simulink model "UAM_Flight_control"  (R2024b)
settings: Solver=FixedStepAuto  StartTime=0.0  StopTime=inf  RelTol=1e-3  EnableMultiTasking=on
undefined symbols (not defined in the file): CityMission, control, controlParams, ControlSampleTime, Cruise_a, DiscIntNeverNeededParam, Earth, FixedWingMission, flightState, FSState, FWControlParams, FWTrimSpeed, HoverMission, params, position, R_WAYPOINTTRANSITION, TransitionMission, uavParam, Vt, w_trim, WGS84, zGround
libraries: slpidlib x56, simulink x32, uavalgslib x7, robotcorelib x2, simulink_extras x2, mspfiltlib x1, aerolibtransform2 x1
(part 2 of 13)

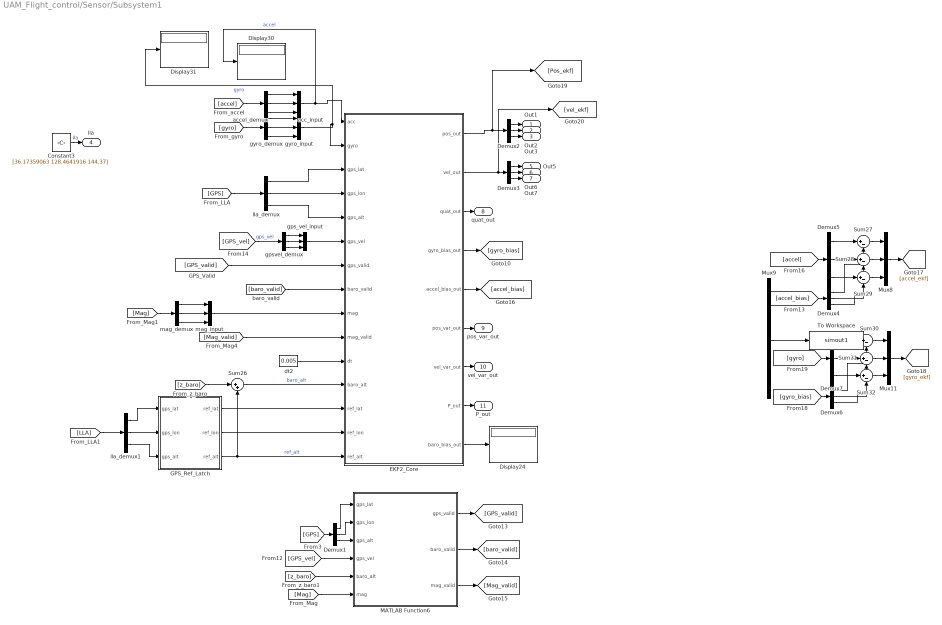
== system UAM_Flight_control/Sensor/Subsystem1 ==
  Constant3 : Constant  Value=[36.17359063 128.4641916 144.37]
  Demux{1..7} (7 alike) : Demux  Outputs=3
  Display24 : Display
  Display30 : Display
  Display31 : Display
  EKF2_Core : Subsystem
  GPS_Ref_Latch : MATLAB Function  TreatAsAtomicUnit=on
  MATLAB Function6 : MATLAB Function  TreatAsAtomicUnit=on
  Mux11 : Mux  Inputs=3
  Mux8 : Mux  Inputs=3
  Mux9 : Mux  Inputs=8
  Sum26 : Sum  Inputs=|++
  Sum{27..32} (6 alike) : Sum  Inputs=|+-
  To Workspace : ToWorkspace  VariableName=simout1  SaveFormat=Structure With Time  SampleTime=-1
  acc_input : Mux  Inputs=3
  accel_demux : Demux  Outputs=3
  dt2 : Constant  Value=0.005
  gps_vel_input : Mux  Inputs=3
  gpsvel_demux : Demux  Outputs=3
  gyro_demux : Demux  Outputs=3
  gyro_input : Mux  Inputs=3
  lla_demux : Demux  Outputs=3
  lla_demux1 : Demux  Outputs=3
  mag_demux : Demux  Outputs=3
  mag_input : Mux  Inputs=3
  Out1 : Outport
  Out2 : Outport  Port=2
  Out3 : Outport  Port=3
  lla : Outport  Port=4
  Out5 : Outport  Port=5
  Out6 : Outport  Port=6
  Out7 : Outport  Port=7
  quat_out : Outport  Port=8
  pos_var_out : Outport  Port=9
  vel_var_out : Outport  Port=10
  P_out : Outport  Port=11
  wires:
  GPS_Ref_Latch/1(ref_lat) -> EKF2_Core/13(ref_lat)
  [Mag] -> MATLAB Function6/6(mag)
  [GPS_vel] -> MATLAB Function6/4(gps_vel)
  EKF2_Core/3(quat_out) -> quat_out/1
  gpsvel_demux/3 -> gps_vel_input/3
  [Mag] -> mag_demux/1
  lla_demux1/3 -> GPS_Ref_Latch/3(gps_alt)
  acc_input/1 -> Display30/1, EKF2_Core/1(acc)  "accel"
  [accel] -> accel_demux/1
  GPS_Ref_Latch/3(ref_alt) -> Sum26/2, EKF2_Core/15(ref_alt)  "ref_alt"
  gyro_demux/3 -> gyro_input/3
  mag_demux/1 -> mag_input/1
  Sum26/1 -> EKF2_Core/12(baro_alt)  "baro_alt"
  gyro_demux/1 -> gyro_input/1
  EKF2_Core/7(vel_var_out) -> vel_var_out/1
  Demux1/2 -> MATLAB Function6/2(gps_lon)
  mag_input/1 -> EKF2_Core/9(mag)
  EKF2_Core/9(baro_bias_out) -> Display24/1
  [baro_valid] -> EKF2_Core/8(baro_valid)
  [LLA] -> lla_demux1/1
  EKF2_Core/5(accel_bias_out) -> [accel_bias]
  Demux2/3 -> Out3/1
  [gyro] -> gyro_demux/1
  MATLAB Function6/1(gps_valid) -> [GPS_valid]
  Demux2/2 -> Out2/1
  [z_baro] -> MATLAB Function6/5(baro_alt)
  [GPS_vel] -> gpsvel_demux/1  "gps_vel"
  gpsvel_demux/1 -> gps_vel_input/1
  Demux2/1 -> Out1/1
  GPS_Ref_Latch/2(ref_lon) -> EKF2_Core/14(ref_lon)
  lla_demux1/1 -> GPS_Ref_Latch/1(gps_lat)
  gyro_demux/2 -> gyro_input/2
  mag_demux/2 -> mag_input/2
  lla_demux/1 -> EKF2_Core/3(gps_lat)
  MATLAB Function6/2(baro_valid) -> [baro_valid]
  [GPS] -> lla_demux/1
  accel_demux/3 -> acc_input/3
  Demux1/1 -> MATLAB Function6/1(gps_lat)
  Demux1/3 -> MATLAB Function6/3(gps_alt)
  MATLAB Function6/3(mag_valid) -> [Mag_valid]
  dt2/1 -> EKF2_Core/11(dt)
  [Mag_valid] -> EKF2_Core/10(mag_valid)
  EKF2_Core/6(pos_var_out) -> pos_var_out/1
  Demux3/2 -> Out6/1
  [z_baro] -> Sum26/1
  accel_demux/1 -> acc_input/1
  [GPS_valid] -> EKF2_Core/7(gps_valid)
  EKF2_Core/2(vel_out) -> [vel_ekf], Demux3/1
  Constant3/1 -> lla/1  "lla"
  lla_demux1/2 -> GPS_Ref_Latch/2(gps_lon)
  gps_vel_input/1 -> EKF2_Core/6(gps_vel)
  accel_demux/2 -> acc_input/2
  gyro_input/1 -> EKF2_Core/2(gyro), Display31/1  "gyro"
  [GPS] -> Demux1/1
  lla_demux/3 -> EKF2_Core/5(gps_alt)
  EKF2_Core/1(pos_out) -> [Pos_ekf], Demux2/1
  EKF2_Core/8(P_out) -> P_out/1
  EKF2_Core/4(gyro_bias_out) -> [gyro_bias]
  lla_demux/2 -> EKF2_Core/4(gps_lon)
  gpsvel_demux/2 -> gps_vel_input/2
  mag_demux/3 -> mag_input/3
  Demux3/3 -> Out7/1
  Demux3/1 -> Out5/1
  Sum31/1 -> Mux11/2
  Demux6/3 -> Sum32/2
  Mux11/1 -> [gyro_ekf]
  [gyro] -> Demux7/1
  Mux8/1 -> [accel_ekf]
  Sum30/1 -> Mux11/1
  Sum29/1 -> Mux8/3
  Sum28/1 -> Mux8/2
  Demux5/1 -> Sum27/1
  Mux9/1 -> To Workspace/1
  Demux6/1 -> Sum30/2
  Demux7/1 -> Sum30/1
  [accel_bias] -> Demux4/1
  Demux7/2 -> Sum31/1
  [gyro_bias] -> Demux6/1
  [accel] -> Demux5/1
  Demux4/2 -> Sum28/2
  Demux5/2 -> Sum28/1
  Demux7/3 -> Sum32/1
  Demux4/3 -> Sum29/2
  Sum27/1 -> Mux8/1
  Sum32/1 -> Mux11/3
  Demux4/1 -> Sum27/2
  Demux6/2 -> Sum31/2
  Demux5/3 -> Sum29/1

== system UAM_Flight_control/Sensor/Subsystem2 ==
  fcc : Inport
  In2 : Inport  Port=2
  Constant1 : Constant  Value=0
  Gain : Gain  Gain=pi/180
  Gain1 : Gain  Gain=pi/180
  Matrix Concatenate : Concatenate  NumInputs=3  Mode=Multidimensional array  ConcatenateDimension=2
  Product{,1..3} (4 alike) : Product
  Trigonometric Function : Trigonometry
  Trigonometric Function1 : Trigonometry  Operator=cos
  Trigonometric Function2 : Trigonometry  Operator=cos
  Trigonometric Function3 : Trigonometry
  Unary Minus{,1..5} (6 alike) : UnaryMinus
  Vector Concatenate : Concatenate  NumInputs=3
  Vector Concatenate1 : Concatenate  NumInputs=3
  Vector Concatenate2 : Concatenate  NumInputs=3
  Out1 : Outport
  wires:
  Product3/1 -> Unary Minus3/1
  Vector Concatenate/1 -> Matrix Concatenate/1
  Trigonometric Function1/1 -> Vector Concatenate1/2, Product3/2, Product/2, Product2/2
  Unary Minus4/1 -> Vector Concatenate2/3
  Vector Concatenate2/1 -> Matrix Concatenate/3
  Trigonometric Function3/1 -> Unary Minus5/1, Product1/2
  Trigonometric Function/1 -> Product1/1, Unary Minus4/1, Product/1
  Gain/1 -> Trigonometric Function2/1, Trigonometric Function/1
  Product/1 -> Unary Minus/1
  Vector Concatenate1/1 -> Matrix Concatenate/2
  Trigonometric Function2/1 -> Product2/1, Product3/1, Vector Concatenate/3
  fcc/1 -> Gain/1
  Gain1/1 -> Trigonometric Function1/1, Trigonometric Function3/1
  Constant1/1 -> Vector Concatenate1/3
  Unary Minus5/1 -> Vector Concatenate1/1
  In2/1 -> Gain1/1
  Unary Minus2/1 -> Vector Concatenate2/1
  Product2/1 -> Unary Minus2/1
  Product1/1 -> Unary Minus1/1
  Unary Minus/1 -> Vector Concatenate/1
  Unary Minus1/1 -> Vector Concatenate/2
  Unary Minus3/1 -> Vector Concatenate2/2
  Matrix Concatenate/1 -> Out1/1

== system UAM_Flight_control/Controller/Auto1/Blend Scheduler ==
  note: Forward Transition Tilt Mode Manager
  FlightMode : Inport
  States : Inport  Port=2
  MixerCommands : Inport  Port=3
  BTalpha : Subsystem  TreatAsAtomicUnit=on
  Bus Creator : BusCreator  Inputs=5
  Bus Selector1 : BusSelector  OutputSignals=w_phi,w_theta,w_psi,w_z
  Constant : Constant  Value=flightState.Transition
  Constant2 : Constant  Value=0.25*uavParam.geom.mass*9.81
  Constant3 : Constant  Value=FWTrimSpeed
  Constant4 : Constant  Value=FWTrimSpeed
  Constant5 : Constant
  Constant6 : Constant  Value=78.54
  Constant7 : Constant
  Demux : Demux
  FTalpha : Subsystem
  Gain3 : Gain  Gain=0
  Mux : Mux
  Product1 : Product
  Product2 : Product
  Product3 : Product
  Relational Operator : RelationalOperator  Operator===  OutDataTypeStr=boolean  RndMeth=Simplest  InputSameDT=off
  Subtract : Sum  Inputs=+-
  Subtract1 : Sum  Inputs=+-
  Sum1 : Sum  Inputs=|++
  Sum3 : Sum  Inputs=|+-
  Switch : Switch  Criteria=u2 > Threshold  SaturateOnIntegerOverflow=off  InputSameDT=off
  Switch1 : Switch  Criteria=u2 > Threshold  SaturateOnIntegerOverflow=off  InputSameDT=off
  MotorCommands : Outport
  alpha : Outport  Port=2
  FlightState : Outport  Port=3
  wires:
  FlightMode/1 -> Relational Operator/1, FlightState/1
  Relational Operator/1 -> [trigger]
  Bus Selector1/4 -> Sum1/1  "<w_z>"
  Constant2/1 -> Sum1/2
  [liftblending] -> Product2/2
  Mux/1 -> Product2/1
  MixerCommands/1 -> Bus Selector1/1
  Bus Selector1/1 -> Mux/1  "<w_phi>"
  Bus Selector1/2 -> Mux/2  "<w_theta>"
  Bus Selector1/3 -> Mux/3  "<w_psi>"
  Sum1/1 -> Mux/4  "w_z"
  Product2/1 -> Demux/1
  Demux/1 -> Bus Creator/1  "w_phi"
  Demux/2 -> Bus Creator/2  "w_theta"
  Demux/3 -> Bus Creator/3  "w_psi"
  Demux/4 -> Bus Creator/4  "w_z"
  Bus Creator/1 -> MotorCommands/1
  Constant6/1 -> Product1/1
  States/1 -> FTalpha/1(States), BTalpha/1(States)
  Switch/1 -> [liftblending], Subtract1/2
  FTalpha/1(alpha) -> Switch/1
  BTalpha/1(alpha) -> Switch/3
  [trigger] -> Switch/2
  Product1/1 -> Sum3/2
  Sum3/1 -> Switch1/1  "cruise"
  [trigger] -> Switch1/2
  Switch1/1 -> Bus Creator/5  "cruise"
  Constant3/1 -> Gain3/1
  Gain3/1 -> Product3/1
  Constant5/1 -> Subtract/1
  [liftblending] -> Subtract/2
  Subtract/1 -> Product3/2
  Product3/1 -> Switch1/3
  Constant7/1 -> Subtract1/1
  Subtract1/1 -> alpha/1
  Constant/1 -> Relational Operator/2
  [liftblending] -> Product1/2
  Constant4/1 -> Sum3/1

== system UAM_Flight_control/Controller/Auto1/Fixed Wing Controller ==
  States : Inport
  Control Mode : Inport  Port=2
  AAC SP : Inport  Port=3  OutDataTypeStr=Bus: AAC
  FixedWingSP : Inport  Port=4  OutDataTypeStr=Bus: FixedWingCommandBus
  AERT : Inport  Port=5
  In1 : Inport  Port=6
  Actuator Armed : EnablePort
  Subsystem : Subsystem
  Actuator : Outport
  wires:
  States/1 -> Subsystem/1(States)
  Control Mode/1 -> Subsystem/2(Control Mode)
  AAC SP/1 -> Subsystem/3(AAC SP)
  Subsystem/1(Actuator) -> Actuator/1
  AERT/1 -> Subsystem/5(AERT)
  FixedWingSP/1 -> Subsystem/4(FixedWingSP)
  In1/1 -> Subsystem/6(Intransition)

== system UAM_Flight_control/Controller/Auto1/Manual Control ==
  Bus Creator : BusCreator  Inputs=4
  Constant{,1..3} (4 alike) : Constant  Value=0  SampleTime=-1
  AERT : Outport
  wires:
  Constant/1 -> Bus Creator/1  "aileron"
  Constant1/1 -> Bus Creator/2  "throttle"
  Constant2/1 -> Bus Creator/3  "elevator"
  Constant3/1 -> Bus Creator/4  "rudder"
  Bus Creator/1 -> AERT/1

== system UAM_Flight_control/Controller/Auto1/Multicopter Controller ==
  note: Prefilter
  Hover Commands : Inport  OutDataTypeStr=Bus: HoverSPBus
  States : Inport  Port=2
  InTransition : Inport  Port=3
  FlightMode : Inport  Port=4
  " Armed" : EnablePort
  Attitude & Altitude controller : Subsystem
  Demux1 : Demux
  Horizontal Position Control : Subsystem  TreatAsAtomicUnit=on
  Merge : Merge
  Merge1 : Merge
  Mux : Mux  Inputs=3
  NOT1 : Logic  Operator=NOT  IconShape=distinctive  AllPortsSameDT=off  OutDataTypeStr=boolean
  Organize Inputs : Subsystem
  transition controller : Subsystem
  MixerCommands : Outport
  wires:
  Organize Inputs/1(MixerCommands) -> MixerCommands/1
  Demux1/1 -> [XRef]
  [State] -> Horizontal Position Control/3(States)
  Demux1/3 -> [ZRef]
  NOT1/1 -> Horizontal Position Control/Enable
  [XRef] -> Horizontal Position Control/1(XRef)
  [YRef] -> Horizontal Position Control/2(YRef)
  InTransition/1 -> [Transition]
  States/1 -> [State]
  Hover Commands/1 -> Demux1/1
  Demux1/4 -> [YawRef]
  Mux/1 -> Attitude & Altitude controller/1(Ref Attitude)
  [State] -> Attitude & Altitude controller/2(States)
  [ZRef] -> Attitude & Altitude controller/3(Z ref)
  [Transition] -> Attitude & Altitude controller/4(InTransition)
  Attitude & Altitude controller/1(Roll torque cmd) -> Organize Inputs/2(commanded phi torque)
  Attitude & Altitude controller/2(Pitch torque Cmd) -> Organize Inputs/3(commanded theta torque)
  Attitude & Altitude controller/4(commanded thrust) -> Organize Inputs/5(commanded thrust)
  FlightMode/1 -> Attitude & Altitude controller/5(FlightMode)
  Attitude & Altitude controller/3(Yaw torque Cmd) -> Organize Inputs/4(commanded psi torque)
  [Transition] -> NOT1/1, transition controller/Enable
  [YawRef] -> Mux/3
  Demux1/2 -> [YRef]
  Merge/1 -> Mux/1
  Merge1/1 -> Mux/2
  transition controller/1(Rollcmd) -> Merge/2
  transition controller/2(Pitchcmd) -> Merge1/2
  Horizontal Position Control/1(Roll Cmd) -> Merge/1
  Horizontal Position Control/2(Pitch Cmd) -> Merge1/1

== system UAM_Flight_control/Controller/Auto1/Scheduler ==
  MotorCommands : Inport
  FlightState : Inport  Port=2  OutDataTypeStr=Enum: flightState
  FixedWingActuators : Inport  Port=3
  " Armed" : EnablePort
  FixedWingScheduler : Subsystem
  Subsystem : Subsystem
  MotorActuatorCommands : Outport  OutputWhenDisabled=reset  InitialOutput=0
  CtrlSurfaceCommands : Outport  Port=2  OutDataTypeStr=Bus: FixedWingCtrlBus  OutputWhenDisabled=reset  InitialOutput=0  VectorParamsAs1DForOutWhenUnconnected=off
  wires:
  FixedWingScheduler/1(ActuatorControls) -> CtrlSurfaceCommands/1, Subsystem/2(FixedWingActuators)
  FlightState/1 -> Subsystem/1(FlightState), FixedWingScheduler/1(FlightState)
  Subsystem/1(ActuatorControls) -> MotorActuatorCommands/1
  MotorCommands/1 -> Subsystem/3(MotorCommands)
  FixedWingActuators/1 -> FixedWingScheduler/2(FixedWingActuators)

== system UAM_Flight_control/Controller/Emergency/Blend Scheduler ==
  FlightMode : Inport
  States : Inport  Port=2
  Constant : Constant  Value=flightState.Transition
  Constant1 : Constant  Value=flightState.BackTransition
  Discrete-Time Integrator : DiscreteIntegrator  gainval=0.01  SampleTime=-1  ICPrevOutput=DiscIntNeverNeededParam  ICPrevScaledInput=DiscIntNeverNeededParam
  Gain : Gain
  Gain1 : Gain  Gain=-1
  Relational Operator : RelationalOperator  Operator===  OutDataTypeStr=boolean  RndMeth=Simplest  InputSameDT=off
  Relational Operator1 : RelationalOperator  Operator===  OutDataTypeStr=boolean  RndMeth=Simplest  InputSameDT=off
  Saturation : Saturate  UpperLimit=1  LowerLimit=0  OutDataTypeStr=double
  Sum : Sum  Inputs=|++
  Terminator : Terminator
  alpha : Outport
  FlightState : Outport  Port=2
  wires:
  FlightMode/1 -> Relational Operator1/1, Relational Operator/1, FlightState/1
  Gain/1 -> Sum/1
  Gain1/1 -> Sum/2
  Sum/1 -> Discrete-Time Integrator/1
  Discrete-Time Integrator/1 -> Saturation/1
  Saturation/1 -> alpha/1  "a"
  States/1 -> Terminator/1
  Constant/1 -> Relational Operator/2
  Relational Operator/1 -> Gain/1
  Constant1/1 -> Relational Operator1/2
  Relational Operator1/1 -> Gain1/1

== system UAM_Flight_control/Controller/Emergency/FixedWing Controller ==
  States : Inport
  Control Mode : Inport  Port=2
  RC : Inport  Port=3
  Actuator Armed : EnablePort
  Subsystem : Subsystem
  Actuator : Outport
  wires:
  States/1 -> Subsystem/1(States)
  Control Mode/1 -> Subsystem/2(Control Mode)
  Subsystem/1(Actuator) -> Actuator/1
  RC/1 -> Subsystem/3(RC)

== system UAM_Flight_control/Controller/Emergency/Scheduler ==
  MotorCommands : Inport
  BlendingSchedule : Inport  Port=2
  FlightState : Inport  Port=3  OutDataTypeStr=Enum: flightState
  TransitionDone : Inport  Port=4
  BackTransitionDone : Inport  Port=5
  FixedWingActuators : Inport  Port=6  OutDataTypeStr=Bus: FixedWingCtrlBus
  Actuator Armed : EnablePort
  FixedWingScheduler : Subsystem
  Subsystem : Subsystem
  MotorActuatorCommands : Outport  OutputWhenDisabled=reset  InitialOutput=0
  CtrlSurfaceCommands : Outport  Port=2  OutDataTypeStr=Bus: FixedWingCtrlBus  OutputWhenDisabled=reset  InitialOutput=0  VectorParamsAs1DForOutWhenUnconnected=off
  wires:
  FixedWingScheduler/1(ActuatorControls) -> CtrlSurfaceCommands/1, Subsystem/2(FixedWingActuators)
  FlightState/1 -> Subsystem/1(FlightState), FixedWingScheduler/1(FlightState)
  BlendingSchedule/1 -> Subsystem/4(BlendingSchedule)
  Subsystem/1(ActuatorControls) -> MotorActuatorCommands/1
  MotorCommands/1 -> Subsystem/3(MotorCommands)
  FixedWingActuators/1 -> FixedWingScheduler/2(FixedWingActuators)
  TransitionDone/1 -> Subsystem/5(TransitionDone), FixedWingScheduler/3(TransitionDone)
  BackTransitionDone/1 -> Subsystem/6(BackTransitionDone)

== system UAM_Flight_control/Controller/Emergency/multicopter Controller ==
  RC : Inport
  States : Inport  Port=2
  Actuator Armed : EnablePort
  Attitude & Altitude controller : Subsystem
  Demux : Demux  Outputs=10
  Mux1 : Mux  Inputs=3
  Organize Inputs : Subsystem
  Terminator{,1..6} (7 alike) : Terminator
  MixerCommands : Outport
  wires:
  Demux/6 -> Terminator2/1
  Organize Inputs/1(MixerCommands) -> MixerCommands/1
  Demux/2 -> Organize Inputs/1(forward command), Mux1/2
  Demux/5 -> Terminator1/1
  Attitude & Altitude controller/3(Yaw torque Cmd) -> Organize Inputs/4(commanded psi torque)
  States/1 -> Attitude & Altitude controller/2(States)
  Demux/4 -> Mux1/3
  Attitude & Altitude controller/1(Roll torque cmd) -> Organize Inputs/2(commanded phi torque)
  Attitude & Altitude controller/2(Pitch torque Cmd) -> Organize Inputs/3(commanded theta torque)
  Attitude & Altitude controller/4(commanded thrust) -> Organize Inputs/5(commanded thrust)
  Demux/1 -> Mux1/1
  Mux1/1 -> Attitude & Altitude controller/1(Ref Attitude)
  Demux/3 -> Terminator/1
  RC/1 -> Demux/1
  Demux/7 -> Terminator3/1
  Demux/8 -> Terminator4/1
  Demux/9 -> Terminator5/1
  Demux/10 -> Terminator6/1

== system UAM_Flight_control/Controller/Manual/Blend Scheduler ==
  FlightMode : Inport
  States : Inport  Port=2
  Constant : Constant  Value=flightState.Transition
  Constant1 : Constant  Value=flightState.BackTransition
  Discrete-Time Integrator : DiscreteIntegrator  gainval=0.01  SampleTime=-1  ICPrevOutput=DiscIntNeverNeededParam  ICPrevScaledInput=DiscIntNeverNeededParam
  Gain : Gain
  Gain1 : Gain  Gain=-1
  Relational Operator : RelationalOperator  Operator===  OutDataTypeStr=boolean  RndMeth=Simplest  InputSameDT=off
  Relational Operator1 : RelationalOperator  Operator===  OutDataTypeStr=boolean  RndMeth=Simplest  InputSameDT=off
  Saturation : Saturate  UpperLimit=1  LowerLimit=0  OutDataTypeStr=double
  Sum : Sum  Inputs=|++
  Terminator : Terminator
  alpha : Outport
  FlightState : Outport  Port=2
  wires:
  FlightMode/1 -> Relational Operator1/1, Relational Operator/1, FlightState/1
  Gain/1 -> Sum/1
  Gain1/1 -> Sum/2
  Sum/1 -> Discrete-Time Integrator/1
  Discrete-Time Integrator/1 -> Saturation/1
  Saturation/1 -> alpha/1  "a"
  States/1 -> Terminator/1
  Constant/1 -> Relational Operator/2
  Relational Operator/1 -> Gain/1
  Constant1/1 -> Relational Operator1/2
  Relational Operator1/1 -> Gain1/1

== system UAM_Flight_control/Controller/Manual/FixedWing Controller ==
  States : Inport
  Control Mode : Inport  Port=2
  RC : Inport  Port=3
  Actuator Armed : EnablePort
  Subsystem : Subsystem
  Actuator : Outport
  wires:
  States/1 -> Subsystem/1(States)
  Control Mode/1 -> Subsystem/2(Control Mode)
  Subsystem/1(Actuator) -> Actuator/1
  RC/1 -> Subsystem/3(RC)

== system UAM_Flight_control/Controller/Manual/Scheduler ==
  MotorCommands : Inport
  BlendingSchedule : Inport  Port=2
  FlightState : Inport  Port=3  OutDataTypeStr=Enum: flightState
  TransitionDone : Inport  Port=4
  BackTransitionDone : Inport  Port=5
  FixedWingActuators : Inport  Port=6  OutDataTypeStr=Bus: FixedWingCtrlBus
  Actuator Armed : EnablePort
  FixedWingScheduler : Subsystem
  Subsystem : Subsystem
  MotorActuatorCommands : Outport  OutputWhenDisabled=reset  InitialOutput=0
  CtrlSurfaceCommands : Outport  Port=2  OutDataTypeStr=Bus: FixedWingCtrlBus  OutputWhenDisabled=reset  InitialOutput=0  VectorParamsAs1DForOutWhenUnconnected=off
  wires:
  FixedWingScheduler/1(ActuatorControls) -> CtrlSurfaceCommands/1, Subsystem/2(FixedWingActuators)
  FlightState/1 -> Subsystem/1(FlightState), FixedWingScheduler/1(FlightState)
  BlendingSchedule/1 -> Subsystem/4(BlendingSchedule)
  Subsystem/1(ActuatorControls) -> MotorActuatorCommands/1
  MotorCommands/1 -> Subsystem/3(MotorCommands)
  FixedWingActuators/1 -> FixedWingScheduler/2(FixedWingActuators)
  TransitionDone/1 -> Subsystem/5(TransitionDone), FixedWingScheduler/3(TransitionDone)
  BackTransitionDone/1 -> Subsystem/6(BackTransitionDone)

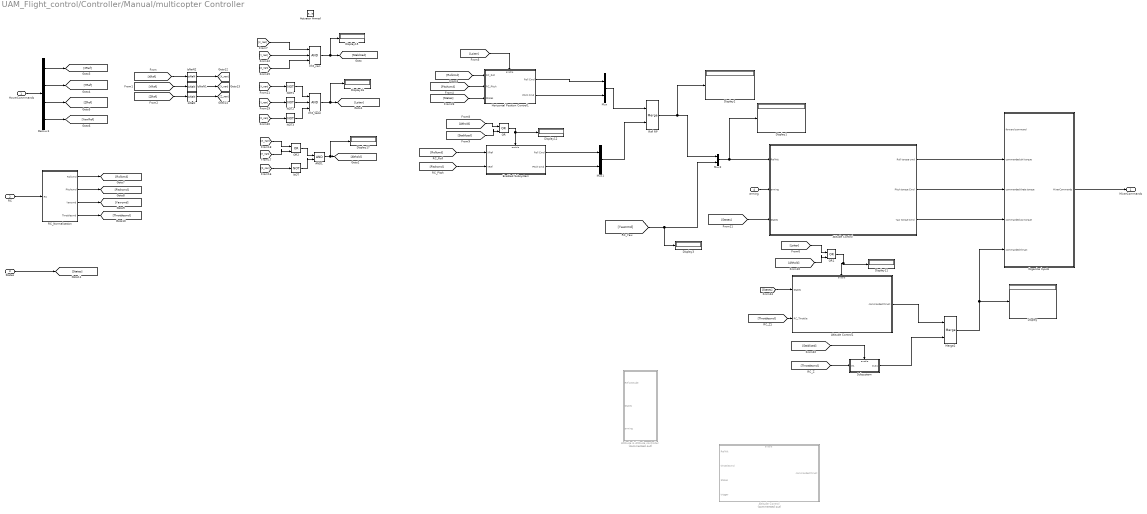
== system UAM_Flight_control/Controller/Manual/multicopter Controller ==
  HoverConmmands : Inport
  RC : Inport  Port=2
  States : Inport  Port=3
  arming : Inport  Port=4
  Actuator Armed : EnablePort
  AND1 : Logic  IconShape=distinctive  AllPortsSameDT=off  OutDataTypeStr=boolean
  Altitude Control : Subsystem  Commented=on
  Altitude Control1 : Subsystem
  Atitude Control : Subsystem
  Attitude & Altitude controller : Subsystem  Commented=on
  Demux1 : Demux
  Display{,1..3,11..12,15..17} (9 alike) : Display
  Enabled Subsystem : Subsystem  TreatAsAtomicUnit=on
  Horizontal Position Control1 : Subsystem  TreatAsAtomicUnit=on
  IsNaN : RelationalOperator  Operator=isNaN  OutDataTypeStr=boolean  RndMeth=Simplest  InputSameDT=off
  IsNaN1 : RelationalOperator  Operator=isNaN  OutDataTypeStr=boolean  RndMeth=Simplest  InputSameDT=off
  IsNaN2 : RelationalOperator  Operator=isNaN  OutDataTypeStr=boolean  RndMeth=Simplest  InputSameDT=off
  Merge2 : Merge
  Mux : Mux  Inputs=2
  Mux1 : Mux  Inputs=2
  Mux2 : Mux  Inputs=2
  NOT{,1..3} (4 alike) : Logic  Operator=NOT  IconShape=distinctive  AllPortsSameDT=off  OutDataTypeStr=boolean
  OR : Logic  Operator=OR  IconShape=distinctive  AllPortsSameDT=off  OutDataTypeStr=boolean
  OR1 : Logic  Operator=OR  IconShape=distinctive  AllPortsSameDT=off  OutDataTypeStr=boolean
  OR2 : Logic  Operator=OR  IconShape=distinctive  AllPortsSameDT=off  OutDataTypeStr=boolean
  Organize Inputs : Subsystem
  RC_Normalization : Subsystem
  Ref RP : Merge
  Subsystem : Subsystem
  XYZ_Valid : Logic  Inputs=3  IconShape=distinctive  AllPortsSameDT=off  OutDataTypeStr=boolean
  XYZ_nan : Logic  Inputs=3  IconShape=distinctive  AllPortsSameDT=off  OutDataTypeStr=boolean
  MixerCommands : Outport
  wires:
  Organize Inputs/1(MixerCommands) -> MixerCommands/1
  HoverConmmands/1 -> Demux1/1
  Demux1/1 -> [XRef]
  Demux1/2 -> [YRef]
  Demux1/3 -> [ZRef]
  Demux1/4 -> [YawRef]
  [XRef] -> IsNaN2/1
  [YRef] -> IsNaN1/1
  [ZRef] -> IsNaN/1
  RC/1 -> RC_Normalization/1(RC)
  RC_Normalization/1(Rollcmd) -> [Rollcmd]
  RC_Normalization/2(Pitchcmd) -> [Pitchcmd]
  RC_Normalization/3(Yawcmd) -> [Yawcmd]
  RC_Normalization/4(Throttlecmd) -> [Throttlecmd]
  [Rollcmd] -> Enabled Subsystem/1(XRef)
  [Pitchcmd] -> Enabled Subsystem/2(YRef)
  Enabled Subsystem/1(Roll Cmd) -> Mux1/1
  Enabled Subsystem/2(Pitch Cmd) -> Mux1/2
  Mux1/1 -> Ref RP/2
  OR/1 -> Enabled Subsystem/Enable, Display12/1
  [Althold] -> OR/1
  [Stablized] -> OR/2
  Ref RP/1 -> Display2/1, Mux2/1
  [Yawcmd] -> Display3/1, Mux2/2
  Mux2/1 -> Atitude Control/1(Ref Att), Display1/1
  arming/1 -> Atitude Control/2(arming)
  States/1 -> [States]
  Atitude Control/1(Roll torque cmd) -> Organize Inputs/2(commanded phi torque)
  Atitude Control/2(Pitch torque Cmd) -> Organize Inputs/3(commanded theta torque)
  Atitude Control/3(Yaw torque Cmd) -> Organize Inputs/4(commanded psi torque)
  [States] -> Atitude Control/3(States)
  Merge2/1 -> Organize Inputs/5(commanded thrust), Display/1
  [Loiter] -> OR1/1
  OR1/1 -> Altitude Control1/Enable, Display11/1
  [Althold] -> OR1/2
  AND1/1 -> Display17/1, [Althold]
  IsNaN2/1 -> [X_nan]
  IsNaN1/1 -> [Y_nan]
  IsNaN/1 -> [Z_nan]
  [X_nan] -> XYZ_nan/1
  [Y_nan] -> XYZ_nan/2
  [Z_nan] -> XYZ_nan/3
  [Z_nan] -> NOT/1
  NOT/1 -> AND1/2
  OR2/1 -> AND1/1
  [X_nan] -> OR2/1
  [Y_nan] -> OR2/2
  [X_nan] -> NOT1/1
  NOT1/1 -> XYZ_Valid/1
  NOT2/1 -> XYZ_Valid/2
  [Y_nan] -> NOT2/1
  [Z_nan] -> NOT3/1
  NOT3/1 -> XYZ_Valid/3
  XYZ_Valid/1 -> Display16/1, [Loiter]
  [Throttlecmd] -> Subsystem/1(In1)
  Subsystem/1(Out1) -> Merge2/2
  [Stablized] -> Subsystem/Enable
  Mux/1 -> Ref RP/1
  XYZ_nan/1 -> Display15/1, [Stablized]
  [States] -> Altitude Control1/1(States)
  [Throttlecmd] -> Altitude Control1/2(RC_Throttle)
  Altitude Control1/1(commanded thrust) -> Merge2/1
  Horizontal Position Control1/2(Pitch Cmd) -> Mux/2
  Horizontal Position Control1/1(Roll Cmd) -> Mux/1
  [States] -> Horizontal Position Control1/3(States)
  [Rollcmd] -> Horizontal Position Control1/1(RC_Roll)
  [Pitchcmd] -> Horizontal Position Control1/2(RC_Pitch)
  [Loiter] -> Horizontal Position Control1/Enable

== system UAM_Flight_control/Flightmode/Auto/Guidance Mode Selector/GuidanceLogic.BackTransition ==
  States : Inport  OutDataTypeStr=Bus: GuidanceStates
  Action Port : ActionPort
      settings: CopyFcn=Stateflow.SLINSF.SimulinkMan.removeBlockPreDeleteFcn  PreDeleteFcn=Stateflow.SLINSF.SimulinkMan.unsafePredeleteFcn
  Bus Creator1 : BusCreator  Inputs=3  OutDataTypeStr=Bus: innerLoopCmdsBus  NonVirtualBus=on
  Bus Selector : BusSelector  OutputSignals=Xe
  Constant : Constant  Value=0
  Constant1 : Constant  Value=0
  Constant2 : Constant  Value=0
  Data Type Conversion : DataTypeConversion  OutDataTypeStr=uint8  SaturateOnIntegerOverflow=off  RndMeth=Floor
  Gain : Gain
  Status : Outport
  InnerLoopCmds : Outport  Port=2  OutDataTypeStr=Bus: innerLoopCmdsBus
  wires:
  States/1 -> Bus Selector/1
  Bus Selector/1 -> Gain/1  "<Xe>"
  Bus Creator1/1 -> InnerLoopCmds/1
  Constant1/1 -> Bus Creator1/2  "HeadingCmd"
  Constant2/1 -> Bus Creator1/3  "YawCmd"
  Data Type Conversion/1 -> Status/1
  Gain/1 -> Bus Creator1/1  "LAP"
  Constant/1 -> Data Type Conversion/1

== system UAM_Flight_control/Flightmode/Auto/Guidance Mode Selector/GuidanceLogic.FIXED_WING_ORBIT.ORBIT ==
  ToWP : Inport  OutDataTypeStr=Bus: UAVPathManagerBus
  States : Inport  Port=2
  Action Port : ActionPort
      settings: CopyFcn=Stateflow.SLINSF.SimulinkMan.removeBlockPreDeleteFcn  PreDeleteFcn=Stateflow.SLINSF.SimulinkMan.unsafePredeleteFcn
  Abs1 : Abs  SaturateOnIntegerOverflow=off
  Bus Creator : BusCreator  Inputs=5  OutDataTypeStr=Bus: AAC  NonVirtualBus=on
      settings: InheritFromInputs=off
  Bus Selector : BusSelector  OutputSignals=position,params
  Bus Selector1 : BusSelector  OutputSignals=Xe,course  OutputAsBus=on
  Bus to Vector : BusToVector
  Constant : Constant  Value=control.cruiseSpeed
  Constant1 : Constant  Value=0
  Data Type Conversion : DataTypeConversion  OutDataTypeStr=uint8  SaturateOnIntegerOverflow=off  RndMeth=Floor
  Lookahead Distance : Constant  Value=control.L1  OutDataTypeStr=double
  Relational Operator : RelationalOperator  Operator=>  OutDataTypeStr=boolean  RndMeth=Simplest  InputSameDT=off
  Selector : Selector  InputPortWidth=3  IndexOptions=Index vector (dialog)  Indices=3  OutputSizes=1
  Selector1 : Selector  InputPortWidth=4  IndexOptions=Index vector (dialog)  Indices=2  OutputSizes=1
  Selector2 : Selector  InputPortWidth=4  IndexOptions=Index vector (dialog)  Indices=1  OutputSizes=1
  Selector3 : Selector  InputPortWidth=4  IndexOptions=Index vector (dialog)  Indices=3  OutputSizes=1
  Terminator{,1..3} (4 alike) : Terminator
  UAV Orbit Follower : uavalgslib/Orbit Follower  UAVType=fixed-wing  MinOrbitRadius=control.turningRadius  MinLookaheadDistance=control.L1  ExternalReset=none  ShowCrossTrackErrorOutput=off  ShowNumTurnsOutput=on  SimulateUsing=Code generation
  Unary Minus : UnaryMinus
  Status : Outport
  aacSP : Outport  Port=2
  wires:
  Bus to Vector/1 -> UAV Orbit Follower/1
  Selector2/1 -> UAV Orbit Follower/3
  Bus Selector/1 -> UAV Orbit Follower/2, Selector/1  "<position>"
  ToWP/1 -> Bus Selector/1
  Bus Selector/2 -> Selector1/1, Selector3/1, Selector2/1  "<params>"
  Selector3/1 -> Relational Operator/2
  Relational Operator/1 -> Data Type Conversion/1
  UAV Orbit Follower/4 -> Terminator/1
  UAV Orbit Follower/5 -> Terminator1/1
  Bus Selector1/1 -> Bus to Vector/1
  States/1 -> Bus Selector1/1
  UAV Orbit Follower/1 -> Terminator2/1  "LAP"
  Lookahead Distance/1 -> UAV Orbit Follower/5, Bus Creator/4  "L1"
  Bus Creator/1 -> aacSP/1
  UAV Orbit Follower/2 -> Bus Creator/3  "course"
  Constant/1 -> Bus Creator/1  "airspeed"
  Unary Minus/1 -> Bus Creator/2  "altitude"
  UAV Orbit Follower/3 -> Terminator3/1  "YawCmd"
  Selector/1 -> Unary Minus/1
  UAV Orbit Follower/6 -> Abs1/1
  Abs1/1 -> Relational Operator/1
  Selector1/1 -> UAV Orbit Follower/4
  Constant1/1 -> Bus Creator/5  "climbrate"
  Data Type Conversion/1 -> Status/1

== system UAM_Flight_control/Flightmode/Auto/Guidance Mode Selector/GuidanceLogic.FIXED_WING_WAYPOINT.WAYPOINT ==
  note: This subsystem selects a lookahead point on the path and provides a desired course. Desired course is later converted to desired lateral acceleration (and roll setpoint)
  States : Inport  OutDataTypeStr=Bus: GuidanceStates
  ToWP : Inport  Port=2  OutDataTypeStr=Bus: UAVPathManagerBus
  FromWP : Inport  Port=3  OutDataTypeStr=Bus: UAVPathManagerBus
  Action Port : ActionPort
      settings: CopyFcn=Stateflow.SLINSF.SimulinkMan.removeBlockPreDeleteFcn  PreDeleteFcn=Stateflow.SLINSF.SimulinkMan.unsafePredeleteFcn
  Bus Creator : BusCreator  Inputs=5  OutDataTypeStr=Bus: AAC  NonVirtualBus=on
      settings: InheritFromInputs=off
  Bus Selector : BusSelector  OutputSignals=Xe,course  OutputAsBus=on
  Bus Selector1 : BusSelector  OutputSignals=position
  Bus Selector2 : BusSelector  OutputSignals=position
  Bus to Vector : BusToVector
  Constant : Constant  Value=control.cruiseSpeed
  Constant1 : Constant  Value=0
  Data Type Conversion : DataTypeConversion  SaturateOnIntegerOverflow=off  RndMeth=Floor
  Display{,2..4} (4 alike) : Display
  Lookahead Distance : Constant  Value=control.L1*15  OutDataTypeStr=double
  MATLAB Function : MATLAB Function  TreatAsAtomicUnit=on
  MATLAB Function1 : MATLAB Function  Commented=on  TreatAsAtomicUnit=on
  MATLAB Function2 : MATLAB Function  Commented=on  TreatAsAtomicUnit=on
  Scope : Scope
  Terminator : Terminator
  Terminator1 : Terminator
  Terminator2 : Terminator
  Waypoint Follower : uavalgslib/Waypoint Follower  UAVType=fixed-wing  StartFrom=first  TransitionRadiusSource=internal  TransitionRadius=FWControl.transitionRadius  MinLookaheadDistance=control.L1  HoverAtLastWaypoint=off  YawInput=off  ShowCrossTrackErrorOutput=off  ShowStatusOutput=on  SimulateUsing=Code generation
  Status : Outport
  aacSP : Outport  Port=2
  wires:
  Lookahead Distance/1 -> Waypoint Follower/3, Bus Creator/4  "L1"
  Waypoint Follower/1 -> Display4/1, Terminator/1  "LAP"
  Waypoint Follower/3 -> Terminator1/1  "YawCmd"
  Waypoint Follower/4 -> Terminator2/1
  Constant/1 -> Bus Creator/1  "airspeed"
  States/1 -> Bus Selector/1
  Bus Selector/1 -> Bus to Vector/1
  Waypoint Follower/5 -> Scope/1, Data Type Conversion/1
  Data Type Conversion/1 -> Status/1
  Bus Creator/1 -> aacSP/1
  ToWP/1 -> Bus Selector1/1
  FromWP/1 -> Bus Selector2/1
  Bus Selector1/1 -> MATLAB Function/1(toWP)  "<position>"
  Bus Selector2/1 -> MATLAB Function/2(fromWP)  "<position>"
  MATLAB Function/2(alt) -> Bus Creator/2
  Waypoint Follower/2 -> Display/1, Bus Creator/3  "course"
  Constant1/1 -> Bus Creator/5  "climbrate"
  Bus to Vector/1 -> Display3/1, Waypoint Follower/1
  MATLAB Function/1(wps) -> Display2/1, Waypoint Follower/2

== system UAM_Flight_control/Flightmode/Auto/Guidance Mode Selector/GuidanceLogic.ForwardTransition ==
  ToWP : Inport  OutDataTypeStr=Bus: UAVPathManagerBus
  FromWP : Inport  Port=2  OutDataTypeStr=Bus: UAVPathManagerBus
  Action Port : ActionPort
      settings: CopyFcn=Stateflow.SLINSF.SimulinkMan.removeBlockPreDeleteFcn  PreDeleteFcn=Stateflow.SLINSF.SimulinkMan.unsafePredeleteFcn
  Bus Creator : BusCreator  Inputs=5  OutDataTypeStr=Bus: AAC  NonVirtualBus=on
      settings: InheritFromInputs=off
  Bus Creator1 : BusCreator  Inputs=3  OutDataTypeStr=Bus: innerLoopCmdsBus  NonVirtualBus=on
  Bus Selector1 : BusSelector  OutputSignals=position
  Bus Selector2 : BusSelector  OutputSignals=position
  Constant : Constant  Value=0
  Constant1 : Constant  Value=0
  Constant2 : Constant  Value=0
  Constant3 : Constant  Value=[0 0 0]
  Data Type Conversion : DataTypeConversion  OutDataTypeStr=uint8  SaturateOnIntegerOverflow=off  RndMeth=Floor
  MATLAB Function : MATLAB Function  TreatAsAtomicUnit=on
  Switch : Switch  Criteria=u2 > Threshold  SaturateOnIntegerOverflow=off  InputSameDT=off
  Terminator : Terminator
  Status : Outport
  InnerLoopCmds : Outport  Port=2  OutDataTypeStr=Bus: innerLoopCmdsBus
  aacSP : Outport  Port=3
  wires:
  Bus Creator1/1 -> InnerLoopCmds/1
  Constant1/1 -> Bus Creator1/2  "HeadingCmd"
  Constant2/1 -> Bus Creator1/3  "YawCmd"
  Data Type Conversion/1 -> Status/1
  Constant/1 -> Data Type Conversion/1
  Constant3/1 -> Bus Creator1/1  "LAP"
  FromWP/1 -> Bus Selector2/1
  Bus Selector1/1 -> MATLAB Function/1(toWP)  "<position>"
  Bus Selector2/1 -> MATLAB Function/2(fromWP)  "<position>"
  ToWP/1 -> Bus Selector1/1
  Bus Creator/1 -> aacSP/1
  MATLAB Function/1(wps) -> Terminator/1
  MATLAB Function/2(alt) -> Bus Creator/2  "alt"

== system UAM_Flight_control/Flightmode/Auto/Guidance Mode Selector/GuidanceLogic.Land.Descend ==
  ToWP : Inport  OutDataTypeStr=Bus: UAVPathManagerBus
  Ground : Inport  Port=2
  Pose : Inport  Port=3
  FromWP : Inport  Port=4  OutDataTypeStr=Bus: UAVPathManagerBus
  Action Port : ActionPort
      settings: CopyFcn=Stateflow.SLINSF.SimulinkMan.removeBlockPreDeleteFcn  PreDeleteFcn=Stateflow.SLINSF.SimulinkMan.unsafePredeleteFcn
  Bus Creator : BusCreator  Inputs=3  OutDataTypeStr=Bus: innerLoopCmdsBus  NonVirtualBus=on
      settings: InheritFromInputs=off
  Bus Selector : BusSelector  OutputSignals=position,params
  Constant : Constant  Value=3
  Constant3 : Constant  Value=0  OutDataTypeStr=uint8
  Hdg Cmd Sat : Saturate  UpperLimit=pi  LowerLimit=-pi
      settings: AttributesFormatString=[%<UpperLimit> %<LowerLimit>]
  MATLAB Function : MATLAB Function  TreatAsAtomicUnit=on
  Mux : Mux  Inputs=2
  Selector : Selector  InputPortWidth=3  IndexOptions=Index vector (dialog)  Indices=[1 2]  OutputSizes=1
  Selector1 : Selector  InputPortWidth=4  IndexOptions=Index vector (dialog)  Indices=1  OutputSizes=1
  Selector3 : Selector  InputPortWidth=4  IndexOptions=Index vector (dialog)  Indices=1  OutputSizes=1
  Waypoint Follower : uavalgslib/Waypoint Follower  UAVType=multirotor  StartFrom=first  TransitionRadiusSource=internal  TransitionRadius=1  MinLookaheadDistance=0.1  HoverAtLastWaypoint=on  YawInput=on  ShowCrossTrackErrorOutput=off  ShowStatusOutput=off  SimulateUsing=Code generation
  Yaw Cmd Sat : Saturate  UpperLimit=pi  LowerLimit=-pi
      settings: AttributesFormatString=[%<UpperLimit> %<LowerLimit>]
  InnerLoopCmds : Outport  OutDataTypeStr=Bus: innerLoopCmdsBus
  Status : Outport  Port=2
  wires:
  Bus Creator/1 -> InnerLoopCmds/1
  Bus Selector/1 -> Selector/1  "<position>"
  Yaw Cmd Sat/1 -> Bus Creator/3  "YawCmd"
  Hdg Cmd Sat/1 -> Bus Creator/2  "HeadingCmd"
  ToWP/1 -> Bus Selector/1
  Selector1/1 -> Yaw Cmd Sat/1
  Selector3/1 -> Hdg Cmd Sat/1
  Selector/1 -> Mux/1  "LAP"
  Bus Selector/2 -> MATLAB Function/3(ToWPParam), Selector1/1, Selector3/1  "<params>"
  Ground/1 -> Mux/2
  Constant3/1 -> Status/1
  Mux/1 -> MATLAB Function/2(ToWPPos)  "LAP"
  FromWP/1 -> MATLAB Function/1(FromWP)
  Pose/1 -> Waypoint Follower/1
  MATLAB Function/1(wps) -> Waypoint Follower/2
  Constant/1 -> Waypoint Follower/3
  Waypoint Follower/1 -> Bus Creator/1  "LAP"

== system UAM_Flight_control/Flightmode/Auto/Guidance Mode Selector/GuidanceLogic.Land.ToLand ==
  Pose : Inport
  ToWP : Inport  Port=2  OutDataTypeStr=Bus: UAVPathManagerBus
  FromWP : Inport  Port=3  OutDataTypeStr=Bus: UAVPathManagerBus
  Action Port : ActionPort
      settings: CopyFcn=Stateflow.SLINSF.SimulinkMan.removeBlockPreDeleteFcn  PreDeleteFcn=Stateflow.SLINSF.SimulinkMan.unsafePredeleteFcn
  Bus Creator1 : BusCreator  Inputs=3  OutDataTypeStr=Bus: innerLoopCmdsBus  NonVirtualBus=on
  Constant : Constant  Value=0  OutDataTypeStr=uint8
  Lookahead Distance : Constant  Value=10  OutDataTypeStr=double
  MATLAB Function : MATLAB Function  TreatAsAtomicUnit=on
  Scope : Scope
  Waypoint Follower : uavalgslib/Waypoint Follower  UAVType=multirotor  StartFrom=first  TransitionRadiusSource=internal  TransitionRadius=1  MinLookaheadDistance=0.1  HoverAtLastWaypoint=on  YawInput=on  ShowCrossTrackErrorOutput=off  ShowStatusOutput=off  SimulateUsing=Code generation
  Status : Outport
  InnerLoopCmds : Outport  Port=2  OutDataTypeStr=Bus: innerLoopCmdsBus
  wires:
  Constant/1 -> Status/1
  MATLAB Function/1(wps) -> Waypoint Follower/2
  Lookahead Distance/1 -> Waypoint Follower/3
  Bus Creator1/1 -> InnerLoopCmds/1
  ToWP/1 -> MATLAB Function/2(ToWP)
  Waypoint Follower/2 -> Bus Creator1/2  "HeadingCmd"
  FromWP/1 -> MATLAB Function/1(FromWP)
  Waypoint Follower/4 -> Scope/1
  Pose/1 -> Waypoint Follower/1
  Waypoint Follower/3 -> Bus Creator1/3  "YawCmd"
  Waypoint Follower/1 -> Bus Creator1/1  "LAP"

== system UAM_Flight_control/Flightmode/Auto/Guidance Mode Selector/GuidanceLogic.Orbit ==
  ToWP : Inport  OutDataTypeStr=Bus: UAVPathManagerBus
  Pose : Inport  Port=2
  Action Port : ActionPort
      settings: CopyFcn=Stateflow.SLINSF.SimulinkMan.removeBlockPreDeleteFcn  PreDeleteFcn=Stateflow.SLINSF.SimulinkMan.unsafePredeleteFcn
  Abs : Abs  SaturateOnIntegerOverflow=off
  Bus Creator : BusCreator  Inputs=3  OutDataTypeStr=Bus: innerLoopCmdsBus  NonVirtualBus=on
  Bus Selector : BusSelector  OutputSignals=position,params
  Data Type Conversion : DataTypeConversion  OutDataTypeStr=uint8  SaturateOnIntegerOverflow=off  RndMeth=Floor
  Lookahead Distance : Constant  Value=5  OutDataTypeStr=double
  Radius : Selector  InputPortWidth=4  IndexOptions=Index vector (dialog)  Indices=[3]  OutputSizes=1
  Relational Operator : RelationalOperator  Operator=>  OutDataTypeStr=boolean  RndMeth=Simplest  InputSameDT=off
  Sign : Signum  ZeroCross=off
  Terminator : Terminator
  Terminator1 : Terminator
  Turns : Selector  InputPortWidth=4  IndexOptions=Index vector (dialog)  Indices=[1]  OutputSizes=1
  UAV Orbit Follower : uavalgslib/Orbit Follower  UAVType=multirotor  MinOrbitRadius=1  MinLookaheadDistance=0.1  ExternalReset=none  ShowCrossTrackErrorOutput=off  ShowNumTurnsOutput=on  SimulateUsing=Code generation
  InnerLoopCmds : Outport  OutDataTypeStr=Bus: innerLoopCmdsBus
  Status : Outport  Port=2
  wires:
  Pose/1 -> UAV Orbit Follower/1
  Lookahead Distance/1 -> UAV Orbit Follower/5
  Abs/1 -> UAV Orbit Follower/3
  Bus Selector/1 -> UAV Orbit Follower/2  "<position>"
  ToWP/1 -> Bus Selector/1
  Bus Creator/1 -> InnerLoopCmds/1
  UAV Orbit Follower/2 -> Bus Creator/2  "HeadingCmd"
  UAV Orbit Follower/3 -> Bus Creator/3  "YawCmd"
  Bus Selector/2 -> Turns/1, Radius/1  "<params>"
  Radius/1 -> Abs/1, Sign/1
  Sign/1 -> UAV Orbit Follower/4
  Relational Operator/1 -> Data Type Conversion/1
  Turns/1 -> Relational Operator/2
  Data Type Conversion/1 -> Status/1
  UAV Orbit Follower/6 -> Relational Operator/1
  UAV Orbit Follower/4 -> Terminator/1
  UAV Orbit Follower/5 -> Terminator1/1
  UAV Orbit Follower/1 -> Bus Creator/1  "LAP"

== system UAM_Flight_control/Flightmode/Auto/Guidance Mode Selector/GuidanceLogic.Takeoff ==
  ToWP : Inport  OutDataTypeStr=Bus: UAVPathManagerBus
  Pose : Inport  Port=2
  Action Port : ActionPort
      settings: CopyFcn=Stateflow.SLINSF.SimulinkMan.removeBlockPreDeleteFcn  PreDeleteFcn=Stateflow.SLINSF.SimulinkMan.unsafePredeleteFcn
  Bus Creator : BusCreator  Inputs=3  OutDataTypeStr=Bus: innerLoopCmdsBus  NonVirtualBus=on
      settings: InheritFromInputs=off
  Bus Selector : BusSelector  OutputSignals=position,params
  Constant : Constant  Value=0  OutDataTypeStr=uint8
  Constant1 : Constant  Value=0
  Demux : Demux  Outputs=[2 2]
  Demux1 : Demux  Outputs=[2 1]
  Hdg. Cmd Sat : Saturate  UpperLimit=pi  LowerLimit=-pi
      settings: AttributesFormatString=[%<UpperLimit> %<LowerLimit>]
  Mux : Mux  Inputs=2
  Selector3 : Selector  InputPortWidth=4  IndexOptions=Index vector (dialog)  Indices=1  OutputSizes=1
  Terminator : Terminator
  Terminator1 : Terminator
  Yaw Cmd Sat : Saturate  UpperLimit=pi  LowerLimit=-pi
      settings: AttributesFormatString=[%<UpperLimit> %<LowerLimit>]
  InnerLoopCmds : Outport  OutDataTypeStr=Bus: innerLoopCmdsBus
  Status : Outport  Port=2
  wires:
  Hdg. Cmd Sat/1 -> Bus Creator/2  "HeadingCmd"
  Bus Creator/1 -> InnerLoopCmds/1
  Constant/1 -> Status/1
  Pose/1 -> Demux/1
  Yaw Cmd Sat/1 -> Bus Creator/3  "YawCmd"
  ToWP/1 -> Bus Selector/1
  Bus Selector/2 -> Selector3/1  "<params>"
  Demux/1 -> Mux/1
  Bus Selector/1 -> Demux1/1  "<position>"
  Demux/2 -> Terminator/1
  Demux1/1 -> Terminator1/1
  Selector3/1 -> Hdg. Cmd Sat/1
  Constant1/1 -> Yaw Cmd Sat/1
  Demux1/2 -> Mux/2
  Mux/1 -> Bus Creator/1  "LAP"

== system UAM_Flight_control/Flightmode/Auto/Guidance Mode Selector/GuidanceLogic.WP ==
  FromWP : Inport  OutDataTypeStr=Bus: UAVPathManagerBus
  Pose : Inport  Port=2
  ToWP : Inport  Port=3  OutDataTypeStr=Bus: UAVPathManagerBus
  Action Port : ActionPort
      settings: CopyFcn=Stateflow.SLINSF.SimulinkMan.removeBlockPreDeleteFcn  PreDeleteFcn=Stateflow.SLINSF.SimulinkMan.unsafePredeleteFcn
  Back Transition Guard : Subsystem
  Bus Creator : BusCreator  Inputs=3  OutDataTypeStr=Bus: innerLoopCmdsBus  NonVirtualBus=on
  Bus Creator1 : BusCreator  Inputs=1
  Bus Creator2 : BusCreator  Inputs=3
  Bus Selector : BusSelector  OutputSignals=position
  Constant1 : Constant  Value=2
  Data Type Conversion : DataTypeConversion  OutDataTypeStr=uint8  SaturateOnIntegerOverflow=off  RndMeth=Floor
  Data Type Conversion1 : DataTypeConversion  OutDataTypeStr=double  SaturateOnIntegerOverflow=off  RndMeth=Floor
  Data Type Conversion2 : DataTypeConversion  OutDataTypeStr=double  SaturateOnIntegerOverflow=off  RndMeth=Floor
  Demux : Demux  Outputs=3
  Dist2WP : Subsystem
  Lookahead Distance : Constant  OutDataTypeStr=double
  MATLAB Function : MATLAB Function  TreatAsAtomicUnit=on
  Relational Operator : RelationalOperator  OutDataTypeStr=boolean  RndMeth=Simplest  InputSameDT=off
  Scope : Scope
  Selector : Selector  InputPortWidth=3  IndexOptions=Index vector (dialog)  Indices=3  OutputSizes=1
  Terminator1 : Terminator
  Waypoint Follower : uavalgslib/Waypoint Follower  UAVType=multirotor  StartFrom=closest  TransitionRadiusSource=internal  TransitionRadius=R_WAYPOINTTRANSITION*3  MinLookaheadDistance=0.1  HoverAtLastWaypoint=on  YawInput=on  ShowCrossTrackErrorOutput=off  ShowStatusOutput=off  SimulateUsing=Code generation
  Yaw Cmd Sat : Saturate  UpperLimit=pi  LowerLimit=-pi
      settings: AttributesFormatString=[%<UpperLimit> %<LowerLimit>]
  InnerLoopCmds : Outport  OutDataTypeStr=Bus: innerLoopCmdsBus
  Status : Outport  Port=2
  wires:
  Data Type Conversion/1 -> Status/1
  Bus Creator/1 -> InnerLoopCmds/1
  ToWP/1 -> Dist2WP/3(ToWP), Bus Selector/1, MATLAB Function/2(ToWP)
  MATLAB Function/1(wps) -> Waypoint Follower/2
  Waypoint Follower/2 -> Bus Creator/2  "HeadingCmd"
  Waypoint Follower/4 -> Scope/1
  Dist2WP/1(Dist) -> Relational Operator/2
  FromWP/1 -> Back Transition Guard/2(FromWP)
  Relational Operator/1 -> Data Type Conversion/1
  Back Transition Guard/1(PrevWP) -> Dist2WP/2(FromWP), MATLAB Function/1(FromWP)
  Pose/1 -> Back Transition Guard/1(Poses), Waypoint Follower/1, Dist2WP/1(Pose)
  Lookahead Distance/1 -> Waypoint Follower/3
  Waypoint Follower/3 -> Yaw Cmd Sat/1  "YawCmd"
  Yaw Cmd Sat/1 -> Bus Creator/3  "YawCmd"
  Constant1/1 -> Relational Operator/1
  Bus Creator1/1 -> Data Type Conversion1/1  "LAP"
  Waypoint Follower/1 -> Demux/1  "LAP"
  Demux/3 -> Terminator1/1
  Data Type Conversion1/1 -> Selector/1  "LAP"
  Selector/1 -> Bus Creator2/3  "Z"
  Demux/1 -> Bus Creator2/1  "X"
  Demux/2 -> Bus Creator2/2  "Y"
  Bus Creator2/1 -> Data Type Conversion2/1  "LAP"
  Data Type Conversion2/1 -> Bus Creator/1  "LAP"
  Bus Selector/1 -> Bus Creator1/1  "<position>"

== system UAM_Flight_control/GNC/Guidance/Auto ==
  note: Ground : 해발고도 기준, 착륙 지점 고도
  Pose : Inport
  Mission : Inport  Port=2  OutDataTypeStr=Bus: UAVPathManagerBus
  isModeDone : Inport  Port=3
  LandingStates : Inport  Port=4
  States : Inport  Port=5
  Ground : Inport  Port=6
  Action Port : ActionPort  ActionPortLabel=case [ Auto ]:
  Bus Creator : BusCreator  Inputs=6  OutDataTypeStr=Bus: GNCplan
  Bus Creator1 : BusCreator  Inputs=3  OutDataTypeStr=Bus: UAVPathManagerBus  NonVirtualBus=on
  Bus Selector : BusSelector  OutputSignals=mode
  Bus Selector1 : BusSelector  OutputSignals=target
  Compare To Constant : simulink/Logic and Bit Operations/Compare To Constant  relop===  const=1  OutDataTypeStr=boolean
  Compare To Constant1 : simulink/Logic and Bit Operations/Compare To Constant  relop=>=  const=3.0  OutDataTypeStr=boolean
  Constant : Constant  Value=0  OutDataTypeStr=uint8
  Constant1 : Constant  Value=[0,0,0]  OutDataTypeStr=double
  Constant2 : Constant  OutDataTypeStr=uint8
  Constant3 : Constant  Value=[0;0;0;0]
  Goto : Goto  Commented=on  GotoTag=landingState
  IC : InitialCondition
  Logical Operator : Logic  Operator=OR  Inputs=1  AllPortsSameDT=off  OutDataTypeStr=boolean
  Path Manager : uavalgslib/Path Manager  UAVType=multirotor  LoiterRadius=25  dataType=double  inputBusName='UAVPathManagerBus'  SimulateUsing=Code generation
  Reshape : Reshape  OutputDimensionality=Customize  OutputDimensions=[3 1]
  Selector : Selector  InputPortWidth=2  IndexOptions=Index vector (dialog)  Indices=1  OutputSizes=1
  Selector1 : Selector  InputPortWidth=2  IndexOptions=Index vector (dialog)  Indices=2  OutputSizes=1
  Switch : Switch  Criteria=u2 > Threshold  SaturateOnIntegerOverflow=off  InputSameDT=off
  GNCPlan : Outport  OutDataTypeStr=Bus: GNCplan
  wires:
  IC/1 -> Bus Creator/1  "mode"
  Ground/1 -> Bus Creator/6  "ground"
  Selector1/1 -> Bus Creator/3  "FromWP"
  States/1 -> Bus Selector1/1, Bus Creator/5  "states"
  Bus Creator/1 -> GNCPlan/1
  Selector/1 -> Bus Selector/1, Switch/3  "ToWP"
  Path Manager/1 -> Selector/1, Selector1/1
  Constant/1 -> Path Manager/4
  Constant1/1 -> Path Manager/5
  Pose/1 -> Bus Creator/4, Path Manager/1  "pose"
  LandingStates/1 -> Goto/1
  Compare To Constant/1 -> Path Manager/3
  isModeDone/1 -> Compare To Constant/1
  Bus Selector/1 -> IC/1  "<mode>"
  Mission/1 -> Path Manager/2
  Bus Selector1/1 -> Reshape/1, Compare To Constant1/1  "<target>"
  Compare To Constant1/1 -> Logical Operator/1
  Logical Operator/1 -> Switch/2
  Switch/1 -> Bus Creator/2  "ToWP"
  Constant2/1 -> Bus Creator1/1  "mode"
  Constant3/1 -> Bus Creator1/3  "params"
  Reshape/1 -> Bus Creator1/2  "position"
  Bus Creator1/1 -> Switch/1

== system UAM_Flight_control/GNC/Guidance/Emergency ==
  pose : Inport
  states : Inport  Port=2
  ground : Inport  Port=3
  Action Port : ActionPort  ActionPortLabel=case [ Emergecny ]:
  Bus Creator : BusCreator  Inputs=6  OutDataTypeStr=Bus: GNCplan
  Constant1 : Constant  Value=struct('mode', uint8(0), 'position', zeros(3,1), 'params', zeros(4,1))  OutDataTypeStr=Bus: UAVPathManagerBus
  Constant2 : Constant  Value=struct('mode', uint8(0), 'position', zeros(3,1), 'params', zeros(4,1))  OutDataTypeStr=Bus: UAVPathManagerBus
  Constant3 : Constant  Value=0  OutDataTypeStr=uint8
  GNCPlan : Outport  OutDataTypeStr=Bus: GNCplan
  wires:
  pose/1 -> Bus Creator/4  "pose"
  Bus Creator/1 -> GNCPlan/1
  Constant1/1 -> Bus Creator/2  "ToWP"
  Constant2/1 -> Bus Creator/3  "FromWP"
  ground/1 -> Bus Creator/6  "ground"
  states/1 -> Bus Creator/5  "states"
  Constant3/1 -> Bus Creator/1  "mode"

== system UAM_Flight_control/GNC/Guidance/Switch Case Action Subsystem ==
  pose : Inport
  states : Inport  Port=2
  ground : Inport  Port=3
  Action Port : ActionPort  ActionPortLabel=case [ Manual ]:
  Bus Creator : BusCreator  Inputs=6  OutDataTypeStr=Bus: GNCplan
  Constant1 : Constant  Value=struct('mode', uint8(0), 'position', zeros(3,1), 'params', zeros(4,1))  OutDataTypeStr=Bus: UAVPathManagerBus
  Constant2 : Constant  Value=struct('mode', uint8(0), 'position', zeros(3,1), 'params', zeros(4,1))  OutDataTypeStr=Bus: UAVPathManagerBus
  Constant3 : Constant  Value=0  OutDataTypeStr=uint8
  GNCPlan : Outport  OutDataTypeStr=Bus: GNCplan
  wires:
  Bus Creator/1 -> GNCPlan/1
  Constant3/1 -> Bus Creator/1  "mode"
  Constant2/1 -> Bus Creator/3  "FromWP"
  Constant1/1 -> Bus Creator/2  "ToWP"
  pose/1 -> Bus Creator/4  "pose"
  states/1 -> Bus Creator/5  "states"
  ground/1 -> Bus Creator/6  "ground"

== system UAM_Flight_control/GNC/Guidance/UAM POS ==
  UAMStates : Inport  OutDataTypeStr=Bus: StateBus
  Bus Creator : BusCreator  Inputs=5
  Bus Selector : BusSelector  OutputSignals=Xe,Ve
  Demux : Demux  Outputs=3
  Display : Display
  Selector : Selector  InputPortWidth=3  IndexOptions=Index vector (dialog)  Indices=[1]  OutputSizes=1
  Selector1 : Selector  InputPortWidth=3  IndexOptions=Index vector (dialog)  Indices=[2]  OutputSizes=1
  POS : Outport
  wires:
  UAMStates/1 -> Bus Selector/1
  Bus Selector/1 -> Demux/1  "<Xe>"
  Demux/1 -> Bus Creator/1  "x"
  Demux/2 -> Bus Creator/2  "y"
  Demux/3 -> Bus Creator/3  "z"
  Bus Selector/2 -> Selector/1, Selector1/1  "<Ve>"
  Selector/1 -> Bus Creator/4  "vx"
  Selector1/1 -> Bus Creator/5  "vy"
  Bus Creator/1 -> Display/1, POS/1

== system UAM_Flight_control/GNC/Guidance/UAM States ==
  UAMStates : Inport
  Bus Creator : BusCreator  Inputs=8
  Bus Selector : BusSelector  OutputSignals=Euler,pqr,Ve,Xe,course,RotorParameters,RC,target
  States : Outport
  wires:
  UAMStates/1 -> Bus Selector/1
  Bus Creator/1 -> States/1
  Bus Selector/1 -> Bus Creator/1  "<Euler>"
  Bus Selector/2 -> Bus Creator/2  "<pqr>"
  Bus Selector/3 -> Bus Creator/3  "<Ve>"
  Bus Selector/5 -> Bus Creator/5  "<course>"
  Bus Selector/4 -> Bus Creator/4  "<Xe>"
  Bus Selector/6 -> Bus Creator/6  "<RotorParameters>"
  Bus Selector/7 -> Bus Creator/7  "<RC>"
  Bus Selector/8 -> Bus Creator/8  "<target>"

== system UAM_Flight_control/GNC/Navigation/LLA2Local ==
  LLA : Inport
  ve : Inport  Port=2
  Enabled Subsystem : Subsystem  Commented=on  TreatAsAtomicUnit=on
  MATLAB Function : MATLAB Function  TreatAsAtomicUnit=on
  Xe : Outport
  wires:
  LLA/1 -> MATLAB Function/1(LLA)
  ve/1 -> MATLAB Function/2(arming)
  MATLAB Function/1(Xe) -> Xe/1
